simulink model "serial_test"  (R2022a)
settings: Solver=FixedStepAuto  StartTime=0.0  StopTime=10.0  FixedStep=1e-3  RelTol=1e-3  EnableMultiTasking=on
libraries: frdmk64flib x3
settings Model: ExtModeTrigDuration=5  Creator=liaml  LastModifiedBy=liaml
settings OptimizationCC: EnhancedBackFolding=on  PassReuseOutputArgsAs=Individual arguments  ZeroExternalMemoryAtStartup=off  ZeroInternalMemoryAtStartup=off  MaxStackSize=64  OptimizeBlockOrder=speed  DifferentSizesBufferReuse=on  OptimizationCustomize=off  EfficientTunableParamExpr=on
settings DebuggingCC: ParameterTunabilityLossMsg=error
settings HardwareCC: ProdBitPerPointer=32  ProdBitPerSizeT=32  ProdBitPerPtrDiffT=32  ProdLargestAtomicInteger=Long  ProdLargestAtomicFloat=Double  ProdWordSize=32  ProdHWDeviceType=ARM Compatible->ARM Cortex
settings SFSimCC: MATLABDynamicMemAlloc=off
settings RTWCC: SystemTargetFile=ert.tlc  HardwareBoard=NXP FRDM-K64F  TLCOptions="-aInlineSetEventsForThisBaseRateFcn=TLC_FALSE -aSuppressMultiTaskScheduler=TLC_FALSE  -aRateBasedStepFcn=0"  TemplateMakefile=ert_default_tmf  Toolchain=GNU Tools for ARM Embedded Processors
settings CodeAppCC: ForceParamTrailComments=on  IgnoreCustomStorageClasses=off  OperatorAnnotations=on  SimulinkDataObjDesc=on  SFDataObjDesc=on  InsertBlockDesc=on
settings ERTTargetCC: ExtModeTransport=4  ExtModeMexFile=sendToCommService

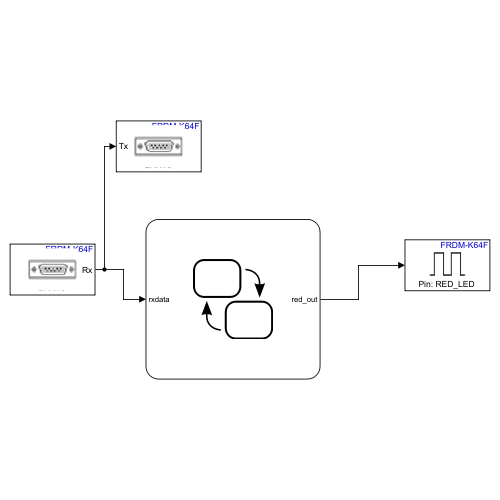
[thumbnail: Simulink's stored preview of the top-level diagram]
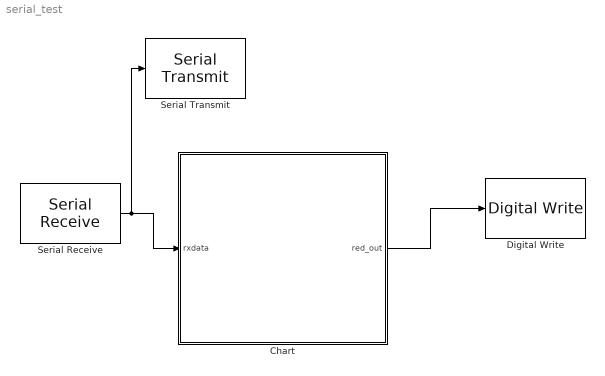
== system serial_test ==
  Chart : Stateflow chart  TreatAsAtomicUnit=on
  Digital Write : frdmk64flib/Digital Write  Whichpin=RED_LED
  Serial Receive : frdmk64flib/Serial Receive  SCIModule=0  Baudrate=uint32(9600)  Parity=None  StopBits=1  HardwareFlowControl=None  ByteOrder=LittleEndian  DataType=int8  DataLength=4  BlockingMode=on  OutputStatus=on  SampleTime=-1
  Serial Transmit : frdmk64flib/Serial Transmit  SCIModule=0  Baudrate=uint32(9600)  Parity=None  StopBits=1  HardwareFlowControl=None  ByteOrder=LittleEndian  BlockingMode=on  OutputStatus=off
  wires:
  Serial Receive/1 -> Serial Transmit/1, Chart/1(rxdata)
  Chart/1(red_out) -> Digital Write/1

== stateflow chart serial_test/Chart ==
  state SET_Params
    entry:
    red_out = 0;
  state Init
    entry:
  state STANDBY
  state Set
    entry:
    red_out = 1;
  SET_Params -> STANDBY
  (default) -> Init
  (junction 41) -> SET_Params [order 2] : [rxdata(1) == hex2dec('5')]
  (junction 41) -> STANDBY [order 3]
  Init -> STANDBY
  STANDBY -> (junction 41)
  (junction 41) -> Set [order 1] : [rxdata(1) == hex2dec('6')]
  Set -> STANDBY
  data: rxdata input; red_out output
